simulink model "sf_variable_size_data"  (Simulink 7.6)
settings: Solver=FixedStepDiscrete  StartTime=0.0  StopTime=5.0  RelTol=1e-3
settings Model: Creator=The MathWorks Inc.
settings DebuggingCC: SolverPrmCheckMsg=none  StrictBusMsg=Warning
settings SFSimCC: SFSimEnableDebug=off  SFSimOverflowDetection=off  SFSimEcho=off  SimParseCustomCode=off

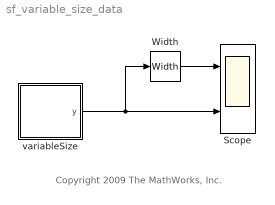
== system sf_variable_size_data ==
  note: Copyright 2009 The MathWorks, Inc.
  Scope : Scope  NumInputPorts=2
      settings: TimeRange=10  YMin=0~0  YMax=8~8
  Width : Width
  variableSize : Stateflow chart  TreatAsAtomicUnit=on
  wires:
  Width/1 -> Scope/1
  variableSize/1(y) -> Scope/2, Width/1

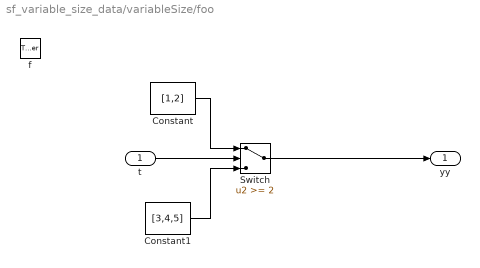
== system sf_variable_size_data/variableSize/foo ==
  t : Inport
  f : TriggerPort  TriggerType=function-call
      settings: CopyFcn=set_param(gcbh,'PreDeleteFcn','')  PreDeleteFcn=Stateflow.SLINSF.SimulinkMan.unsafePredeleteFcn
  Constant : Constant  Value=[1,2]
  Constant1 : Constant  Value=[3,4,5]
  Switch : Switch  Threshold=2  AllowDiffInputSizes=on
  yy : Outport
  wires:
  Constant/1 -> Switch/1
  t/1 -> Switch/2
  Constant1/1 -> Switch/3
  Switch/1 -> yy/1

== stateflow chart variableSize ==
  settings: updateMethod=DISCRETE  sampleTime=.1
  state yy = foo(t) [function]
  (default) -> (junction 4) : {y = foo(t);}
  data: yy function_output double; t function_input double; y output double size=3
